simulink model "Lab01_notes_in_class"  (R2022b)
settings: Solver=VariableStepAuto  StartTime=0.0  StopTime=10.0  RelTol=1e-3
settings Model: Creator=willg  LastModifiedBy=willg

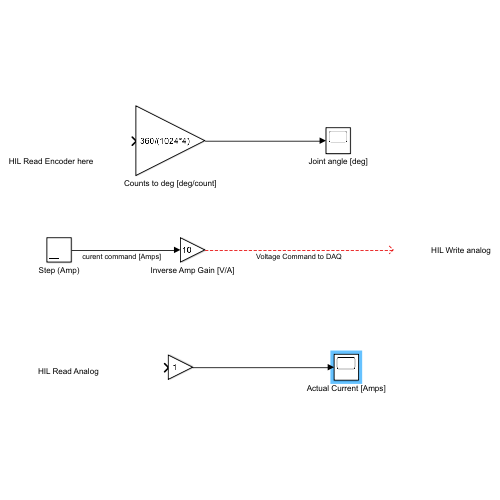
[thumbnail: Simulink's stored preview of the top-level diagram]
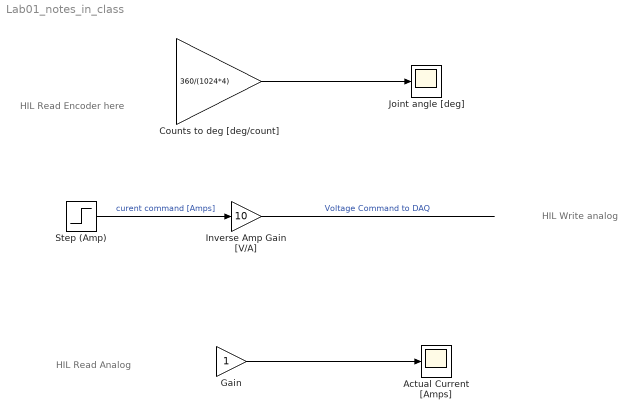
== system Lab01_notes_in_class ==
  note: HIL Read Analog
  note: HIL Write analog
  note: HIL Read Encoder here
  Actual Current [Amps] : Scope
  Counts to deg [deg/count] : Gain  Gain=360/(1024*4)
  Gain : Gain
  Inverse Amp Gain [V/A] : Gain  Gain=10
  Joint angle [deg] : Scope
  Step (Amp) : Step  Time=0  After=0.1  SampleTime=0
  wires:
  Step (Amp)/1 -> Inverse Amp Gain [V/A]/1  "curent command [Amps]"
  Inverse Amp Gain [V/A]/1 -> ?  "Voltage Command to DAQ"
  Counts to deg [deg/count]/1 -> Joint angle [deg]/1
  Gain/1 -> Actual Current [Amps]/1
